simulink library "sensors_S2_design_lib"  (Simulink 6.6)
undefined symbols (not defined in the file or in its folder): AirData, MAG3, POS_hi, POS_lo, SurfacePos, Timestep
libraries: NoiseModel_lib x16, simulink_extras x3, First_Order_Filter_lib x1, Latency_lib x1, simulink x1
settings Model: Creator=amurch  LastModifiedBy=la1032aw  ExtModeAutoUpdateStatusClock=off

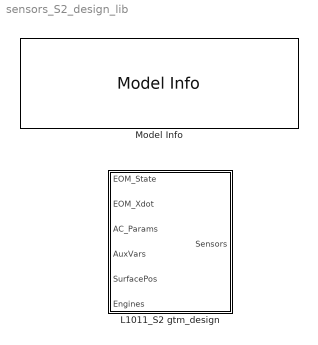
== system sensors_S2_design_lib ==
  L1011_S2 gtm_design : Subsystem
      mask init:
      | if ~exist('MAG3TempComp','var')
      |     appendmws(Cal_params_T2)
      | end
  Model Info : simulink/Model-Wide Utilities/Model Info  SystemSampleTime=-1  InitialBlockCM=None  BlockCM=None  Frame=on  DisplayStringWithTags=|  HorizontalTextAlignment=Center  LeftAlignmentValue=0.5  SourceBlockDiagram=sensors_S2_design_lib  TagMaxNumber=20
      | Sensor Model Library
      | %<ModelVersion>
      | Last modified by %<LastModifiedBy> on %<LastModificationDate>

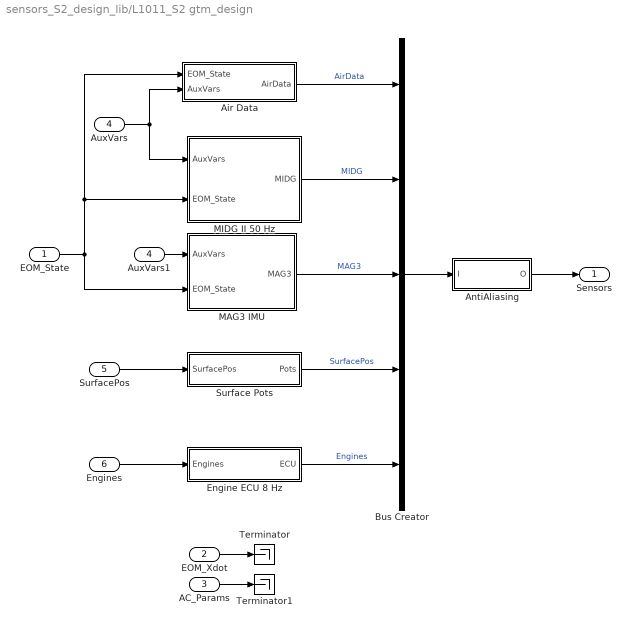
== system sensors_S2_design_lib/L1011_S2 gtm_design ==
  EOM_State : Inport
  EOM_Xdot : Inport  Port=2
  AC_Params : Inport  Port=3
  AuxVars : Inport  Port=4
  SurfacePos : Inport  Port=5
  Engines : Inport  Port=6
  Air Data : Subsystem
  AntiAliasing : Subsystem
  AuxVars1 : InportShadow  Port=4  LatchByCopyingInsideSignal=off
  Bus Creator : BusCreator  Inputs=5
  Engine ECU 8 Hz : Subsystem  SystemSampleTime=round(1/Timestep/8)*Timestep
  MAG3 IMU : Subsystem
  MIDG II 50 Hz : Subsystem  SystemSampleTime=round(1/Timestep/50)*Timestep
  Surface Pots : Subsystem
  Terminator : Terminator
  Terminator1 : Terminator
  Sensors : Outport
  wires:
  EOM_State/1 -> MAG3 IMU/2(EOM_State), MIDG II 50 Hz/2(EOM_State), Air Data/1(EOM_State)
  AuxVars/1 -> MIDG II 50 Hz/1(AuxVars), Air Data/2(AuxVars)
  SurfacePos/1 -> Surface Pots/1(SurfacePos)
  Engines/1 -> Engine ECU 8 Hz/1(Engines)
  MAG3 IMU/1(MAG3) -> Bus Creator/3  "MAG3"
  Engine ECU 8 Hz/1(ECU) -> Bus Creator/5  "Engines"
  Surface Pots/1(Pots) -> Bus Creator/4  "SurfacePos"
  MIDG II 50 Hz/1(MIDG) -> Bus Creator/2  "MIDG"
  Air Data/1(AirData) -> Bus Creator/1  "AirData"
  Bus Creator/1 -> AntiAliasing/1(I)
  AntiAliasing/1(O) -> Sensors/1
  EOM_Xdot/1 -> Terminator/1
  AC_Params/1 -> Terminator1/1
  AuxVars1/1 -> MAG3 IMU/1(AuxVars)

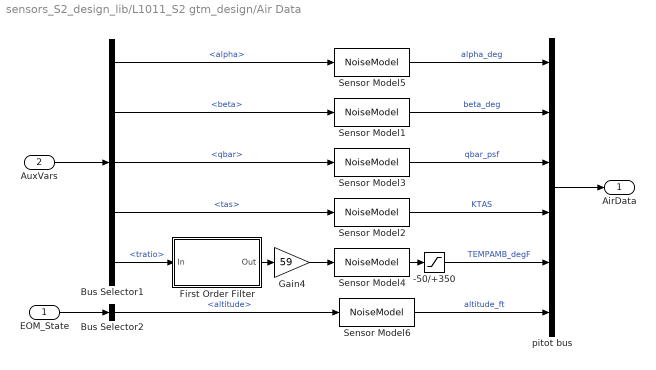
== system sensors_S2_design_lib/L1011_S2 gtm_design/Air Data ==
  EOM_State : Inport
  AuxVars : Inport  Port=2
  -50/+350 : Saturate  UpperLimit=350  LowerLimit=-50
  Bus Selector1 : BusSelector  OutputSignals=alpha,beta,qbar,tas,tratio
  Bus Selector2 : BusSelector  OutputSignals=altitude
  First Order Filter : Subsystem  mask(first order filter){tau=6}
      mask help:
      | __1__
      |  tau s+1
      |
      | First order filter  transfer function
      | with integrator IC = input  at time=0
      | If tau < Simulation Timestep, input is passed through unchanged
      | Simulation timestep must be a variable in the model/base workspace named
      | "Timestep"
      mask Help:
      | This block models a first order filter with the initial condition
      | on the integrator set to the steady state value for constant input.
      | time constant is an input
      mask Display: fprintf('  1\n--------------\n %2.1g s + 1', tau)
  Gain4 : Gain  Gain=59
  Sensor Model1 : NoiseModel_lib/NoiseModel  SystemSampleTime=-1  noise_on=SensorNoise.On  sigma=SensorNoise.beta.Std  seed=878224  bias=SensorNoise.beta.Bias  scf=SensorNoise.beta.Scf
  Sensor Model2 : NoiseModel_lib/NoiseModel  SystemSampleTime=-1  noise_on=SensorNoise.On  sigma=SensorNoise.KTAS.Std  seed=878654  bias=SensorNoise.KTAS.Bias  scf=SensorNoise.KTAS.Scf
  Sensor Model3 : NoiseModel_lib/NoiseModel  SystemSampleTime=-1  noise_on=SensorNoise.On  sigma=SensorNoise.dyn_press.Std  seed=848234  bias=SensorNoise.dyn_press.Bias  scf=SensorNoise.dyn_press.Scf
  Sensor Model4 : NoiseModel_lib/NoiseModel  SystemSampleTime=-1  noise_on=SensorNoise.On  sigma=SensorNoise.tempamb.Std  seed=878634  bias=SensorNoise.tempamb.Bias  scf=SensorNoise.tempamb.Scf
  Sensor Model5 : NoiseModel_lib/NoiseModel  SystemSampleTime=-1  noise_on=SensorNoise.On  sigma=SensorNoise.alpha.Std  seed=278234  bias=SensorNoise.alpha.Bias  scf=SensorNoise.alpha.Scf
  Sensor Model6 : NoiseModel_lib/NoiseModel  SystemSampleTime=-1  noise_on=SensorNoise.On  sigma=SensorNoise.baro_alt.Std  seed=878654  bias=SensorNoise.baro_alt.Bias  scf=SensorNoise.baro_alt.Scf
  pitot bus : BusCreator  Inputs=6
  AirData : Outport
  wires:
  Bus Selector1/5 -> First Order Filter/1(In)  "<tratio>"
  Sensor Model3/1 -> pitot bus/3  "qbar_psf"
  Bus Selector1/3 -> Sensor Model3/1  "<qbar>"
  pitot bus/1 -> AirData/1
  Gain4/1 -> Sensor Model4/1
  Sensor Model4/1 -> -50/+350/1
  -50/+350/1 -> pitot bus/5  "TEMPAMB_degF"
  First Order Filter/1(Out) -> Gain4/1
  Bus Selector1/1 -> Sensor Model5/1  "<alpha>"
  Bus Selector1/2 -> Sensor Model1/1  "<beta>"
  Sensor Model5/1 -> pitot bus/1  "alpha_deg"
  Sensor Model1/1 -> pitot bus/2  "beta_deg"
  Bus Selector1/4 -> Sensor Model2/1  "<tas>"
  Sensor Model2/1 -> pitot bus/4  "KTAS"
  AuxVars/1 -> Bus Selector1/1
  Bus Selector2/1 -> Sensor Model6/1  "<altitude>"
  Sensor Model6/1 -> pitot bus/6  "altitude_ft"
  EOM_State/1 -> Bus Selector2/1

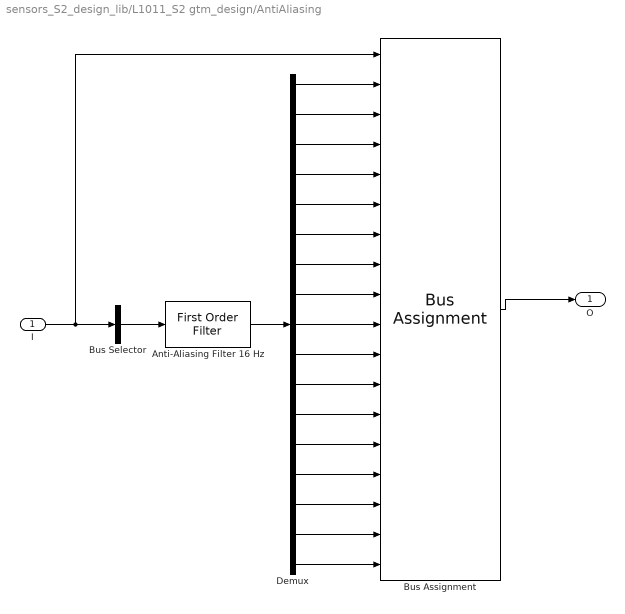
== system sensors_S2_design_lib/L1011_S2 gtm_design/AntiAliasing ==
  I : Inport
  Anti-Aliasing Filter 16 Hz : First_Order_Filter_lib/First Order Filter  SystemSampleTime=-1  tau=1/(32*pi)  timestep=Timestep
  Bus Assignment : BusAssignment  AssignedSignals=AirData.alpha_deg,AirData.beta_deg,AirData.qbar_psf,AirData.KTAS,AirData.TEMPAMB_degF,AirData.altitude_ft,MAG3.p_deg,MAG3.q_deg,MAG3.r_deg,MAG3.Ax_g,MAG3.Ay_g,MAG3.Az_g,SurfacePos.ELL,SurfacePos.ELR,SurfacePos.AILL,SurfacePos.AILR,SurfacePos.RUD
  Bus Selector : BusSelector  OutputSignals=AirData,MAG3,SurfacePos  OutputAsBus=on
  Demux : Demux  Outputs=17
  O : Outport
  wires:
  Bus Assignment/1 -> O/1
  Anti-Aliasing Filter 16 Hz/1 -> Demux/1
  Bus Selector/1 -> Anti-Aliasing Filter 16 Hz/1
  I/1 -> Bus Assignment/1, Bus Selector/1
  Demux/1 -> Bus Assignment/2
  Demux/2 -> Bus Assignment/3
  Demux/3 -> Bus Assignment/4
  Demux/4 -> Bus Assignment/5
  Demux/5 -> Bus Assignment/6
  Demux/6 -> Bus Assignment/7
  Demux/7 -> Bus Assignment/8
  Demux/8 -> Bus Assignment/9
  Demux/9 -> Bus Assignment/10
  Demux/10 -> Bus Assignment/11
  Demux/11 -> Bus Assignment/12
  Demux/12 -> Bus Assignment/13
  Demux/13 -> Bus Assignment/14
  Demux/14 -> Bus Assignment/15
  Demux/15 -> Bus Assignment/16
  Demux/16 -> Bus Assignment/17
  Demux/17 -> Bus Assignment/18

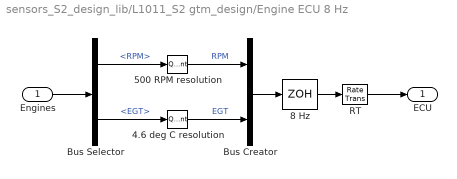
== system sensors_S2_design_lib/L1011_S2 gtm_design/Engine ECU 8 Hz ==
  Engines : Inport
  4.6 deg C resolution : Quantizer  QuantizationInterval=4.6
  500 RPM resolution : Quantizer  QuantizationInterval=500
  8 Hz : ZeroOrderHold  SampleTime=round(1/Timestep/8)*Timestep
  Bus Creator : BusCreator  Inputs=2
  Bus Selector : BusSelector  OutputSignals=RPM,EGT
  RT : RateTransition
  ECU : Outport
  wires:
  Engines/1 -> Bus Selector/1
  4.6 deg C resolution/1 -> Bus Creator/2  "EGT"
  500 RPM resolution/1 -> Bus Creator/1  "RPM"
  Bus Selector/1 -> 500 RPM resolution/1  "<RPM>"
  RT/1 -> ECU/1
  Bus Creator/1 -> 8 Hz/1
  8 Hz/1 -> RT/1
  Bus Selector/2 -> 4.6 deg C resolution/1  "<EGT>"

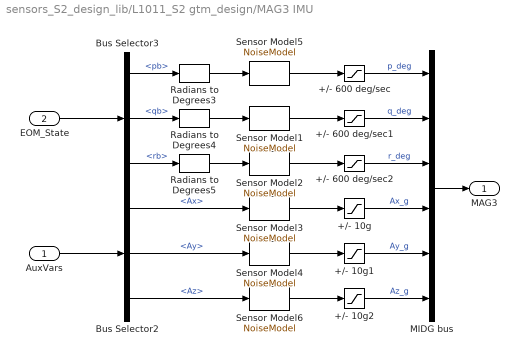
== system sensors_S2_design_lib/L1011_S2 gtm_design/MAG3 IMU ==
  AuxVars : Inport
  EOM_State : Inport  Port=2
  +/- 10g : Saturate  UpperLimit=10  LowerLimit=-10
  +/- 10g1 : Saturate  UpperLimit=10  LowerLimit=-10
  +/- 10g2 : Saturate  UpperLimit=10  LowerLimit=-10
  +/- 600 deg/sec : Saturate  UpperLimit=600  LowerLimit=-600
  +/- 600 deg/sec1 : Saturate  UpperLimit=600  LowerLimit=-600
  +/- 600 deg/sec2 : Saturate  UpperLimit=600  LowerLimit=-600
  Bus Selector2 : BusSelector  OutputSignals=Ax,Ay,Az
  Bus Selector3 : BusSelector  OutputSignals=pb,qb,rb
  MIDG bus : BusCreator  Inputs=6
  Radians to Degrees3 : simulink_extras/Transformations/Radians to Degrees  SystemSampleTime=-1
  Radians to Degrees4 : simulink_extras/Transformations/Radians to Degrees  SystemSampleTime=-1
  Radians to Degrees5 : simulink_extras/Transformations/Radians to Degrees  SystemSampleTime=-1
  Sensor Model1 : NoiseModel_lib/NoiseModel  SystemSampleTime=-1  noise_on=SensorNoise.On  sigma=SensorNoise.MAG3.qdeg.Std  seed=871234  bias=SensorNoise.MAG3.qdeg.Bias  scf=SensorNoise.MAG3.qdeg.Scf
  Sensor Model2 : NoiseModel_lib/NoiseModel  SystemSampleTime=-1  noise_on=SensorNoise.On  sigma=SensorNoise.MAG3.rdeg.Std  seed=878134  bias=SensorNoise.MAG3.rdeg.Bias  scf=SensorNoise.MAG3.rdeg.Scf
  Sensor Model3 : NoiseModel_lib/NoiseModel  SystemSampleTime=-1  noise_on=SensorNoise.On  sigma=SensorNoise.MAG3.nxbody.Std  seed=878234  bias=SensorNoise.MAG3.nxbody.Bias  scf=SensorNoise.MAG3.nxbody.Scf
  Sensor Model4 : NoiseModel_lib/NoiseModel  SystemSampleTime=-1  noise_on=SensorNoise.On  sigma=SensorNoise.MAG3.nybody.Std  seed=8782345  bias=SensorNoise.MAG3.nybody.Bias  scf=SensorNoise.MAG3.nybody.Scf
  Sensor Model5 : NoiseModel_lib/NoiseModel  SystemSampleTime=-1  noise_on=SensorNoise.On  sigma=SensorNoise.MAG3.pdeg.Std  seed=878233  bias=SensorNoise.MAG3.pdeg.Bias  scf=SensorNoise.MAG3.pdeg.Scf
  Sensor Model6 : NoiseModel_lib/NoiseModel  SystemSampleTime=-1  noise_on=SensorNoise.On  sigma=SensorNoise.MAG3.nzbody.Std  seed=878236  bias=SensorNoise.MAG3.nzbody.Bias  scf=SensorNoise.MAG3.nzbody.Scf
  MAG3 : Outport
  wires:
  MIDG bus/1 -> MAG3/1
  AuxVars/1 -> Bus Selector2/1
  Sensor Model5/1 -> +/- 600 deg/sec/1
  Sensor Model6/1 -> +/- 10g2/1
  Sensor Model4/1 -> +/- 10g1/1
  Sensor Model3/1 -> +/- 10g/1
  Sensor Model2/1 -> +/- 600 deg/sec2/1
  Sensor Model1/1 -> +/- 600 deg/sec1/1
  Radians to Degrees5/1 -> Sensor Model2/1
  Radians to Degrees4/1 -> Sensor Model1/1
  Radians to Degrees3/1 -> Sensor Model5/1
  Bus Selector2/3 -> Sensor Model6/1  "<Az>"
  Bus Selector2/2 -> Sensor Model4/1  "<Ay>"
  Bus Selector2/1 -> Sensor Model3/1  "<Ax>"
  Bus Selector3/3 -> Radians to Degrees5/1  "<rb>"
  Bus Selector3/2 -> Radians to Degrees4/1  "<qb>"
  Bus Selector3/1 -> Radians to Degrees3/1  "<pb>"
  EOM_State/1 -> Bus Selector3/1
  +/- 600 deg/sec/1 -> MIDG bus/1  "p_deg"
  +/- 600 deg/sec1/1 -> MIDG bus/2  "q_deg"
  +/- 600 deg/sec2/1 -> MIDG bus/3  "r_deg"
  +/- 10g/1 -> MIDG bus/4  "Ax_g"
  +/- 10g1/1 -> MIDG bus/5  "Ay_g"
  +/- 10g2/1 -> MIDG bus/6  "Az_g"

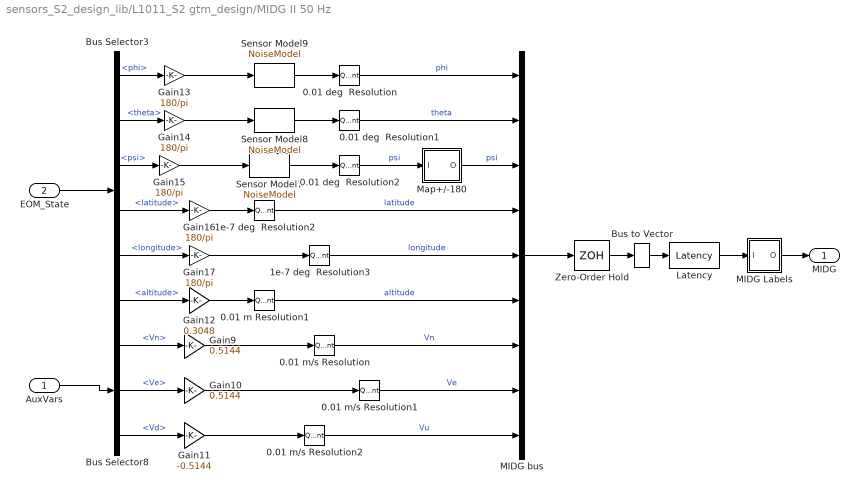
== system sensors_S2_design_lib/L1011_S2 gtm_design/MIDG II 50 Hz ==
  AuxVars : Inport
  EOM_State : Inport  Port=2
  0.01 deg  Resolution : Quantizer  QuantizationInterval=0.01
  0.01 deg  Resolution1 : Quantizer  QuantizationInterval=0.01
  0.01 deg  Resolution2 : Quantizer  QuantizationInterval=0.01
  0.01 m Resolution1 : Quantizer  QuantizationInterval=0.01
  0.01 m/s Resolution : Quantizer  QuantizationInterval=0.01
  0.01 m/s Resolution1 : Quantizer  QuantizationInterval=0.01
  0.01 m/s Resolution2 : Quantizer  QuantizationInterval=0.01
  1e-7 deg  Resolution2 : Quantizer  QuantizationInterval=1e-7
  1e-7 deg  Resolution3 : Quantizer  QuantizationInterval=1e-7
  Bus Selector3 : BusSelector  OutputSignals=phi,theta,psi,latitude,longitude,altitude
  Bus Selector8 : BusSelector  OutputSignals=Vn,Ve,Vd
  Bus to Vector : BusToVector
  Gain10 : Gain  Gain=0.5144
  Gain11 : Gain  Gain=-0.5144
  Gain12 : Gain  Gain=0.3048
  Gain{13..17} (5 alike) : Gain  Gain=180/pi
  Gain9 : Gain  Gain=0.5144
  Latency : Latency_lib/Latency  SystemSampleTime=-1  Latency=.04
  MIDG Labels : Subsystem
  MIDG bus : BusCreator  Inputs=9
  Map+/-180 : Subsystem
  Sensor Model7 : NoiseModel_lib/NoiseModel  SystemSampleTime=-1  noise_on=SensorNoise.On  sigma=SensorNoise.MIDG.psi.Std  seed=878232  bias=SensorNoise.MIDG.psi.Bias  scf=SensorNoise.MIDG.psi.Scf
  Sensor Model8 : NoiseModel_lib/NoiseModel  SystemSampleTime=-1  noise_on=SensorNoise.On  sigma=SensorNoise.MIDG.theta.Std  seed=878231  bias=SensorNoise.MIDG.theta.Bias  scf=SensorNoise.MIDG.theta.Scf
  Sensor Model9 : NoiseModel_lib/NoiseModel  SystemSampleTime=-1  noise_on=SensorNoise.On  sigma=SensorNoise.MIDG.phi.Std  seed=878230  bias=SensorNoise.MIDG.phi.Bias  scf=SensorNoise.MIDG.phi.Scf
  Zero-Order Hold : ZeroOrderHold  SampleTime=round(1/Timestep/50)*Timestep
  MIDG : Outport
  wires:
  Bus to Vector/1 -> Latency/1
  0.01 m/s Resolution2/1 -> MIDG bus/9  "Vu"
  Latency/1 -> MIDG Labels/1(I)
  MIDG Labels/1(O) -> MIDG/1
  Map+/-180/1(O) -> MIDG bus/3  "psi"
  AuxVars/1 -> Bus Selector8/1
  Bus Selector3/6 -> Gain12/1  "<altitude>"
  Bus Selector3/5 -> Gain17/1  "<longitude>"
  Bus Selector3/4 -> Gain16/1  "<latitude>"
  Bus Selector8/3 -> Gain11/1  "<Vd>"
  Bus Selector8/2 -> Gain10/1  "<Ve>"
  Bus Selector8/1 -> Gain9/1  "<Vn>"
  Gain17/1 -> 1e-7 deg  Resolution3/1
  Gain16/1 -> 1e-7 deg  Resolution2/1
  Gain15/1 -> Sensor Model7/1
  Gain14/1 -> Sensor Model8/1
  Gain13/1 -> Sensor Model9/1
  MIDG bus/1 -> Zero-Order Hold/1
  0.01 m/s Resolution1/1 -> MIDG bus/8  "Ve"
  0.01 m/s Resolution/1 -> MIDG bus/7  "Vn"
  Gain12/1 -> 0.01 m Resolution1/1
  Gain11/1 -> 0.01 m/s Resolution2/1
  Gain10/1 -> 0.01 m/s Resolution1/1
  Gain9/1 -> 0.01 m/s Resolution/1
  0.01 m Resolution1/1 -> MIDG bus/6  "altitude"
  1e-7 deg  Resolution3/1 -> MIDG bus/5  "longitude"
  1e-7 deg  Resolution2/1 -> MIDG bus/4  "latitude"
  0.01 deg  Resolution2/1 -> Map+/-180/1(I)  "psi"
  0.01 deg  Resolution1/1 -> MIDG bus/2  "theta"
  0.01 deg  Resolution/1 -> MIDG bus/1  "phi"
  Sensor Model9/1 -> 0.01 deg  Resolution/1
  Sensor Model8/1 -> 0.01 deg  Resolution1/1
  Sensor Model7/1 -> 0.01 deg  Resolution2/1
  Bus Selector3/3 -> Gain15/1  "<psi>"
  Bus Selector3/2 -> Gain14/1  "<theta>"
  Bus Selector3/1 -> Gain13/1  "<phi>"
  EOM_State/1 -> Bus Selector3/1
  Zero-Order Hold/1 -> Bus to Vector/1

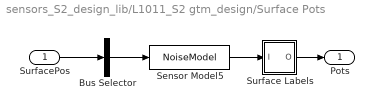
== system sensors_S2_design_lib/L1011_S2 gtm_design/Surface Pots ==
  SurfacePos : Inport
  Bus Selector : BusSelector  OutputSignals=ELL,ELR,AILL,AILR,RUD  OutputAsBus=on
  Sensor Model5 : NoiseModel_lib/NoiseModel  SystemSampleTime=-1  noise_on=SensorNoise.On  sigma=SensorNoise.pots.Std  seed=878239  bias=SensorNoise.pots.Bias  scf=SensorNoise.pots.Scf
  Surface Labels : Subsystem
  Pots : Outport
  wires:
  Surface Labels/1(O) -> Pots/1
  Sensor Model5/1 -> Surface Labels/1(I)
  SurfacePos/1 -> Bus Selector/1
  Bus Selector/1 -> Sensor Model5/1

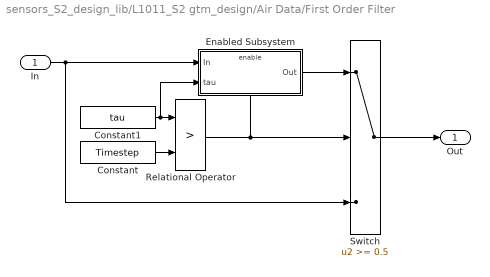
== system sensors_S2_design_lib/L1011_S2 gtm_design/Air Data/First Order Filter ==
  In : Inport
  Constant : Constant  Value=Timestep
  Constant1 : Constant  Value=tau
  Enabled Subsystem : Subsystem  TreatAsAtomicUnit=on
  Relational Operator : RelationalOperator  Operator=>  LogicOutDataTypeMode=Boolean
  Switch : Switch  Threshold=0.5
  Out : Outport
  wires:
  Constant1/1 -> Enabled Subsystem/2(tau), Relational Operator/1
  Enabled Subsystem/1(Out) -> Switch/1
  Switch/1 -> Out/1
  In/1 -> Enabled Subsystem/1(In), Switch/3
  Relational Operator/1 -> Enabled Subsystem/Enable, Switch/2
  Constant/1 -> Relational Operator/2

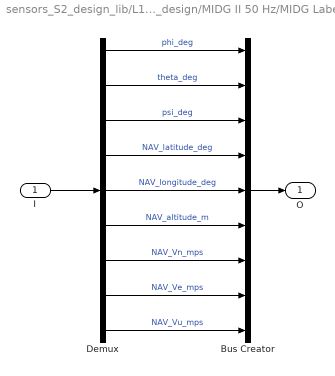
== system sensors_S2_design_lib/L1011_S2 gtm_design/MIDG II 50 Hz/MIDG Labels ==
  I : Inport
  Bus Creator : BusCreator  Inputs=9
  Demux : Demux  Outputs=9
  O : Outport
  wires:
  Demux/9 -> Bus Creator/9  "NAV_Vu_mps"
  Demux/8 -> Bus Creator/8  "NAV_Ve_mps"
  Demux/7 -> Bus Creator/7  "NAV_Vn_mps"
  Demux/6 -> Bus Creator/6  "NAV_altitude_m"
  Demux/5 -> Bus Creator/5  "NAV_longitude_deg"
  Demux/4 -> Bus Creator/4  "NAV_latitude_deg"
  Demux/1 -> Bus Creator/1  "phi_deg"
  Demux/3 -> Bus Creator/3  "psi_deg"
  Demux/2 -> Bus Creator/2  "theta_deg"
  Bus Creator/1 -> O/1
  I/1 -> Demux/1

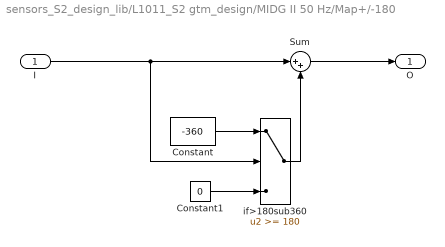
== system sensors_S2_design_lib/L1011_S2 gtm_design/MIDG II 50 Hz/Map+/-180 ==
  I : Inport
  Constant : Constant  Value=-360
  Constant1 : Constant  Value=0
  Sum : Sum  Inputs=|++
  if>180sub360 : Switch  Threshold=180
  O : Outport
  wires:
  Constant/1 -> if>180sub360/1
  Constant1/1 -> if>180sub360/3
  I/1 -> Sum/1, if>180sub360/2
  Sum/1 -> O/1
  if>180sub360/1 -> Sum/2

== system sensors_S2_design_lib/L1011_S2 gtm_design/Surface Pots/Surface Labels ==
  I : Inport
  Bus Creator : BusCreator  Inputs=5
  Demux : Demux  Outputs=5
  O : Outport
  wires:
  I/1 -> Demux/1
  Bus Creator/1 -> O/1
  Demux/1 -> Bus Creator/1  "ELL"
  Demux/2 -> Bus Creator/2  "ELR"
  Demux/3 -> Bus Creator/3  "AILL"
  Demux/4 -> Bus Creator/4  "AILR"
  Demux/5 -> Bus Creator/5  "RUD"

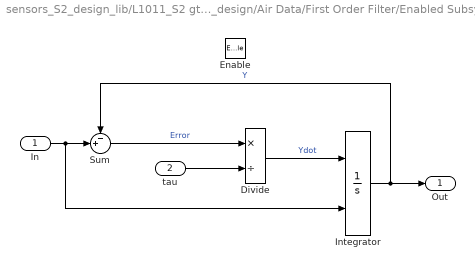
== system sensors_S2_design_lib/L1011_S2 gtm_design/Air Data/First Order Filter/Enabled Subsystem ==
  In : Inport
  tau : Inport  Port=2
  Enable : EnablePort
  Divide : Product  Inputs=*/  OutScaling=2^-10
  Integrator : Integrator  InitialConditionSource=external  UpperSaturationLimit=POS_hi  LowerSaturationLimit=POS_lo
  Sum : Sum  Inputs=-+|  SaturateOnIntegerOverflow=on  InputSameDT=on
  Out : Outport
  wires:
  Sum/1 -> Divide/1  "Error"
  In/1 -> Sum/2, Integrator/2
  Integrator/1 -> Out/1, Sum/1  "Y"
  tau/1 -> Divide/2
  Divide/1 -> Integrator/1  "Ydot"
